simulink model "LinModelMrac"  (R2023b)
settings: Solver=ode23s  StartTime=0.0  StopTime=10.0  RelTol=1e-3
values from neighbouring files (symbols this model uses):
  A_mat = [0,     1,                  0 ... (first row only)    [mracShell.m]    (also in mracShellScaled.m)
  Am = [0,        1,          0 ... (first row only)    [mracShell.m]    (also in mracShellScaled.m)
  B_mat = [0; 0; (-4*beta_e/Ve)*(Kq*Kv)]    [mracShell.m]    (also in mracShellScaled.m)
  Bm = [0; 0; bm3]    [mracShell.m]    (also in mracShellScaled.m)
  gamma_L = gamma_M    (= 1e-12)    [mracShell.m]    (also in mracShellScaled.m = gamma_M)
  gamma_M = 1e-12    [mracShell.m]    (also in mracShellScaled.m = 1 / (norm(B_z)^2 * norm(P_z)))
  P = lyap(Am', Q)    [mracShell.m]
settings Model: Creator=snr  LastModifiedBy=snr

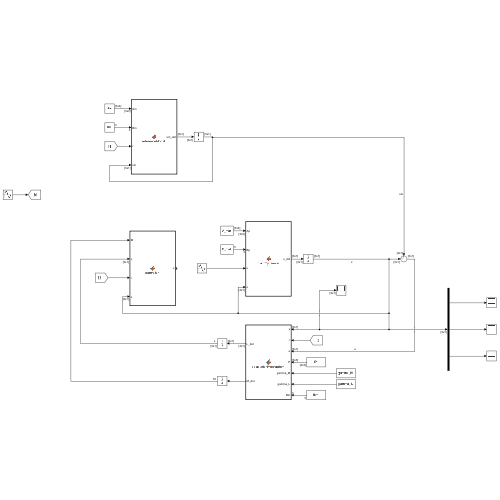
[thumbnail: Simulink's stored preview of the top-level diagram]
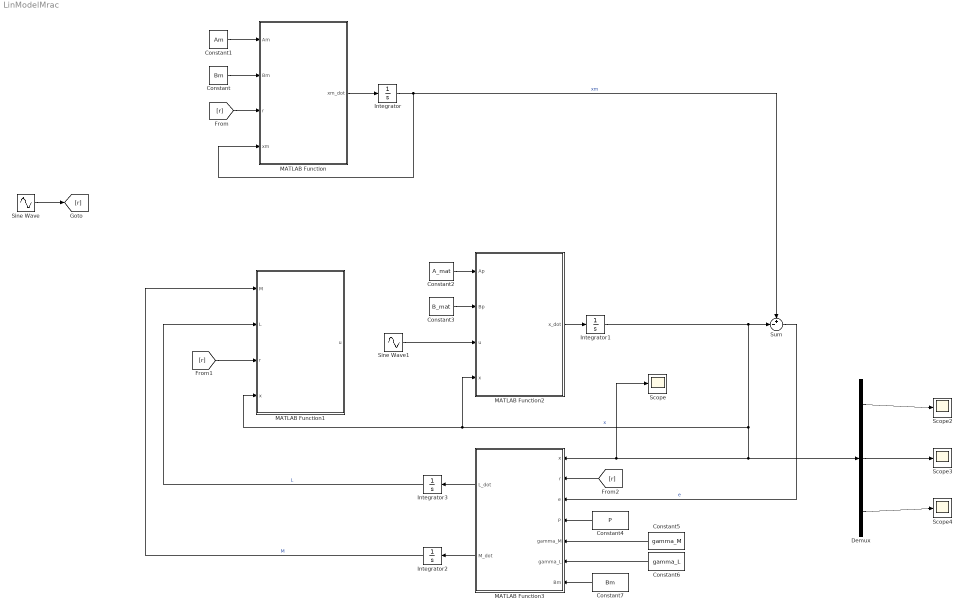
== system LinModelMrac ==
  Constant : Constant  Value=Bm
  Constant1 : Constant  Value=Am
  Constant2 : Constant  Value=A_mat
  Constant3 : Constant  Value=B_mat
  Constant4 : Constant  Value=P
  Constant5 : Constant  Value=gamma_M
  Constant6 : Constant  Value=gamma_L
  Constant7 : Constant  Value=Bm
  Demux : Demux  Outputs=3
  Integrator : Integrator  InitialCondition=[0;0;0]
  Integrator1 : Integrator  InitialCondition=[0;0;0]
  Integrator2 : Integrator
  Integrator3 : Integrator
  MATLAB Function : MATLAB Function  TreatAsAtomicUnit=on
  MATLAB Function1 : MATLAB Function  TreatAsAtomicUnit=on
  MATLAB Function2 : MATLAB Function  TreatAsAtomicUnit=on
  MATLAB Function3 : MATLAB Function  TreatAsAtomicUnit=on
  Scope{,2..4} (4 alike) : Scope
  Sine Wave : Sin  SampleTime=0
  Sine Wave1 : Sin  SampleTime=0
  Sum : Sum  Inputs=+-|
  wires:
  MATLAB Function/1(xm_dot) -> Integrator/1
  Integrator/1 -> Sum/1, MATLAB Function/4(xm)  "xm"
  Sine Wave/1 -> [r]
  [r] -> MATLAB Function/3(r)
  Constant/1 -> MATLAB Function/2(Bm)
  Constant1/1 -> MATLAB Function/1(Am)
  [r] -> MATLAB Function1/3(r)
  MATLAB Function2/1(x_dot) -> Integrator1/1
  Integrator1/1 -> Sum/2, MATLAB Function2/4(x), MATLAB Function1/4(x), Demux/1, Scope/1, MATLAB Function3/1(x)  "x"
  Constant2/1 -> MATLAB Function2/1(Ap)
  Constant3/1 -> MATLAB Function2/2(Bp)
  Constant4/1 -> MATLAB Function3/4(P)
  Constant5/1 -> MATLAB Function3/5(gamma_M)
  Constant6/1 -> MATLAB Function3/6(gamma_L)
  MATLAB Function3/2(M_dot) -> Integrator2/1
  MATLAB Function3/1(L_dot) -> Integrator3/1
  Integrator3/1 -> MATLAB Function1/2(L)  "L"
  Integrator2/1 -> MATLAB Function1/1(M)  "M"
  [r] -> MATLAB Function3/2(r)
  Constant7/1 -> MATLAB Function3/7(Bm)
  Sum/1 -> MATLAB Function3/3(e)  "e"
  Demux/1 -> Scope2/1
  Demux/2 -> Scope3/1
  Demux/3 -> Scope4/1
  Sine Wave1/1 -> MATLAB Function2/3(u)

== matlab function LinModelMrac/MATLAB Function1 ==
  data: M input; u output; L input; r input; x input
function u = controller(M, L, r, x)
    u = M*r - L'*x;
end

% Note
% L -> (1,n)
% x -> (n,1)

% M -> (1,1)
% r -> (1,1)

== matlab function LinModelMrac/MATLAB Function ==
  data: Am input; xm_dot output; Bm input; r input; xm input
function xm_dot = referenceModel(Am, Bm, r, xm)

xm_dot = Am*xm + Bm*r;

== matlab function LinModelMrac/MATLAB Function2 ==
  data: Ap input; Bp input; u input; x_dot output size=[3,1]; x input
function x_dot = plantDynamics(Ap, Bp, u, x)
    x_dot = Ap*x + Bp*u; %[3,3] x [3,1] + [3,1]x[1,1]
end

== matlab function LinModelMrac/MATLAB Function3 ==
  data: x input; r input; e input; L_dot output; P input; gamma_M input; gamma_L input; M_dot output; Bm input
function [L_dot, M_dot] = adaptationMechanism(x, r, e, P, gamma_M, gamma_L, Bm)
    BmT_P_e = Bm'*P*e;   % scalar % [1,3]x[3,3]x[3,1] = [1,1]

    % Adaptasyon (Denklem 8 - DUZELTILMIS ISARET):
    % Makale Eq.(8)'de M_dot isareti (-) yanlis, dogru isaret (+)
    % Lyapunov kaniti: M_dot=+gM*Bm'Pe*r, L_dot=-gL*Bm'Pe*x
    M_dot  = +gamma_M * BmT_P_e * r;    % DUZELTILDI: - degil +
    L_dot  = -gamma_L * BmT_P_e * x;    % dogru: negatif
end

% Note
% L -> (1,n)
% x -> (n,1)

% M -> (1,1)
% r -> (1,1)
